simulink model "Prismatic_Power_Simulink"  (R2021a)
settings: Solver=VariableStepAuto  StartTime=0.0  StopTime=10.0  RelTol=1e-3
libraries: fl_lib x62, nesl_utility x24, fl_ps_legacy_lib x16, ee_lib x7, pid_lib x3, simulink x2
(part 1 of 2)
settings Model: Creator=Shivanshu  LastModifiedBy=Shivanshu

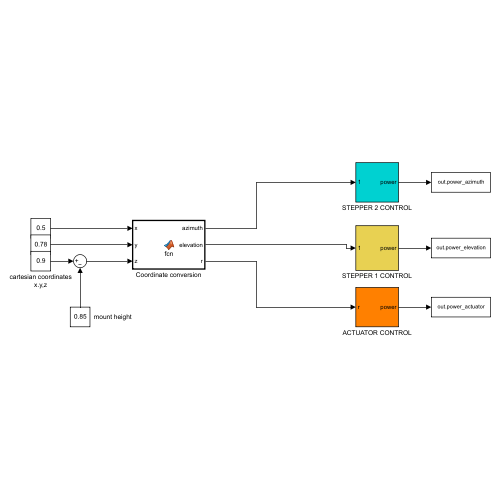
[thumbnail: Simulink's stored preview of the top-level diagram]
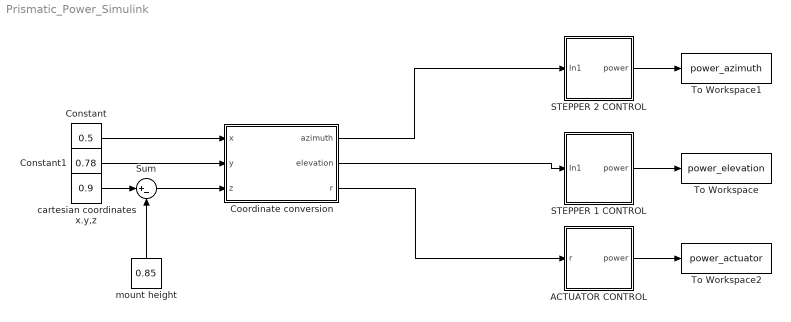
== system Prismatic_Power_Simulink ==
  ACTUATOR CONTROL : Subsystem  RequirementInfo={} %GIDa_0c115b90_ac6e_48f5_b72e_90011be317fb
  Constant : Constant  RequirementInfo={} %GIDa_f342d5e4_ff38_4643_bf1e_b5d7906d0ce5  Value=0.5
  Constant1 : Constant  RequirementInfo={} %GIDa_469f7adb_a8a1_4d2f_b1d5_d7893cc8c779  Value=0.78
  Coordinate conversion : MATLAB Function  RequirementInfo={} %GIDa_592b9090_c388_41e2_bff3_47ffeee67e9d  TreatAsAtomicUnit=on
  STEPPER 1 CONTROL : Subsystem  RequirementInfo={} %GIDa_0e8b4c65_2a77_43a1_8a22_c7e5a5acc945
  STEPPER 2 CONTROL : Subsystem  RequirementInfo={} %GIDa_86f44cae_780d_4682_ad09_b505177498bc
  Sum : Sum  Inputs=|+-
  To Workspace : ToWorkspace  VariableName=power_elevation  SampleTime=-1
  To Workspace1 : ToWorkspace  VariableName=power_azimuth  SampleTime=-1
  To Workspace2 : ToWorkspace  VariableName=power_actuator  SampleTime=-1
  cartesian coordinates x.y,z : Constant  RequirementInfo={} %GIDa_2cf69270_6584_4b69_8bd7_8d40a6ff0831  Value=0.9
  mount height : Constant  Value=0.85
  wires:
  Coordinate conversion/2(elevation) -> STEPPER 1 CONTROL/1(In1)
  Constant1/1 -> Coordinate conversion/2(y)
  Constant/1 -> Coordinate conversion/1(x)
  Coordinate conversion/1(azimuth) -> STEPPER 2 CONTROL/1(In1)
  Coordinate conversion/3(r) -> ACTUATOR CONTROL/1(r)
  Sum/1 -> Coordinate conversion/3(z)
  cartesian coordinates x.y,z/1 -> Sum/1
  mount height/1 -> Sum/2
  ACTUATOR CONTROL/1(power) -> To Workspace2/1
  STEPPER 1 CONTROL/1(power) -> To Workspace/1
  STEPPER 2 CONTROL/1(power) -> To Workspace1/1

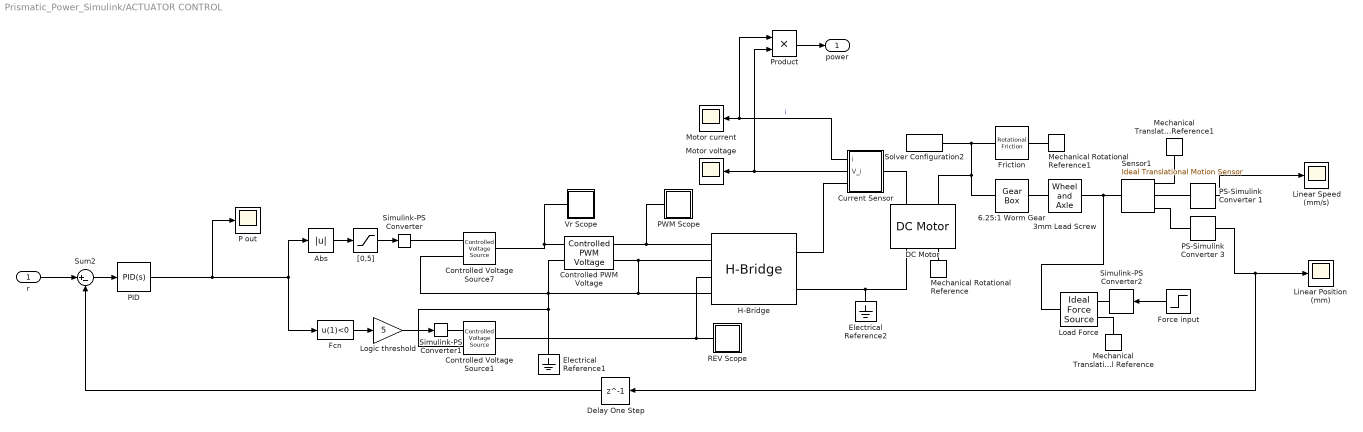
== system Prismatic_Power_Simulink/ACTUATOR CONTROL ==
  r : Inport  RequirementInfo={} %GIDa_01bbb075_66cd_4f10_a905_c743553500a9
  " PID" : pid_lib/PID Controller  RequirementInfo={} %GIDa_487d1a50_046a_4936_a3be_f4ba52b3f77b  Controller=PID  Form=Parallel  TimeDomain=Continuous-time  UseExternalTs=off  SampleTime=-1  IntegratorMethod=Forward Euler  FilterMethod=Forward Euler  ControllerParametersSource=internal  P=50  I=0  D=0  UseFilter=on  N=1  TunerSelectOption=Transfer Function Based (PID Tuner App)  InitialConditionSource=internal  InitialConditionForIntegrator=0  InitialConditionForFilter=0  DifferentiatorICPrevScaledInput=0  ExternalReset=none  TrackingMode=off  Kt=1  LimitOutput=off  SatLimitsSource=internal  UpperSaturationLimit=5  LowerSaturationLimit=-5  LinearizeAsGain=on  AntiWindupMode=back-calculation  Kb=1  POutMin=[]  POutMax=[]  IOutMin=[]  IOutMax=[]  DOutMin=[]  DOutMax=[]  NOutMin=[]  NOutMax=[]  SumOutMin=[]  SumOutMax=[]  SaturationOutMin=[]  SaturationOutMax=[]  PParamMin=[]  PParamMax=[]  IParamMin=[]  IParamMax=[]  DParamMin=[]  DParamMax=[]  NParamMin=[]  NParamMax=[]  KbParamMin=[]  KbParamMax=[]  KtParamMin=[]  KtParamMax=[]  KbOutMin=[]  KbOutMax=[]  KtOutMin=[]  KtOutMax=[]  IntegratorOutMin=[]  IntegratorOutMax=[]  FilterOutMin=[]  FilterOutMax=[]  SumI1OutMin=[]  SumI1OutMax=[]  SumI2OutMin=[]  SumI2OutMax=[]  SumI3OutMin=[]  SumI3OutMax=[]  SumI4OutMin=[]  SumI4OutMax=[]  SumDOutMin=[]  SumDOutMax=[]  DifferentiatorOutMin=[]  DifferentiatorOutMax=[]  FilterDiffOutCoefMin=[]  FilterDiffOutCoefMax=[]  ReciprocalOutMin=[]  ReciprocalOutMax=[]  SumDenOutMin=[]  SumDenOutMax=[]  SumNumOutMin=[]  SumNumOutMax=[]  DivideOutMin=[]  DivideOutMax=[]  UdiffTsProdOutMin=[]  UdiffTsProdOutMax=[]  NTsProdOutMin=[]  NTsProdOutMax=[]  UintegralTsProdOutMin=[]  UintegralTsProdOutMax=[]  UngainTsProdOutMin=[]  UngainTsProdOutMax=[]  IntegratorContinuousStateAttributes=''  IntegratorStateMustResolveToSignalObject=off  IntegratorRTWStateStorageClass=Auto  FilterContinuousStateAttributes=''  FilterStateMustResolveToSignalObject=off  FilterRTWStateStorageClass=Auto  ParallelPVariant=InternalParameters  IdealPVariant=Disabled  IVariant=InternalParameters  DVariant=InternalParameters  IntegratorVariant=Continuous  SatVariant=Disabled  AWVariant=Passthrough  PCopyVariant=Disabled  TRVariant=Disabled  FdbkBlocksVariant=Forward  IdealPFdbkVariant=Disabled  SatFdbkVariant=Disabled  DerivativeFilterVariant=ContFilter  NVariant=InternalParameters  NCopyVariant=Disabled  FilterICVariant=InternalICsFilter  IntegratorICVariant=InternalICs  ExternalResetVariant=Disabled  TRSumVariant=Passthrough  SumFdbkVariant=Disabled  SumVariant=Sum_PID  TsampFilterVariant=InternalTs  TsampNgainVariant=Passthrough  TsampIntegralVariant=Passthrough  ExternalSaturationOutDataTypeStr=Inherit: Same as second input
  3mm Lead Screw : fl_lib/Mechanical/Mechanisms/Wheel and Axle  RequirementInfo={} %GIDa_63769a3e_da90_4985_9ff6_81674143f087  R=3e-3/(2*pi) m  or=1  t_specify=off  t_priority=High  t=0 N*m  t_nominal_specify=off  t_nominal_unit=N*m  t_nominal_value=1  f_specify=off  f_priority=High  f=0 N  f_nominal_specify=off  f_nominal_unit=N  f_nominal_value=1
  6.25:1 Worm Gear : fl_lib/Mechanical/Mechanisms/Gear Box  RequirementInfo={} %GIDa_72538fa4_a052_4650_b0d0_d2ddea2e6bef  ratio=1  t_in_specify=off  t_in_priority=High  t_in=0 N*m  t_in_nominal_specify=off  t_in_nominal_unit=N*m  t_in_nominal_value=1  t_out_specify=off  t_out_priority=High  t_out=0 N*m  t_out_nominal_specify=off  t_out_nominal_unit=N*m  t_out_nominal_value=1
  Abs : Abs  RequirementInfo={} %GIDa_f6d84932_f9cc_4ae6_b8c7_05faab76c6e2
  Controlled PWM Voltage : ee_lib/Integrated Circuits/Controlled PWM Voltage  RequirementInfo={} %GIDa_27007e47_f5f5_44e8_a6b6_33ad898611cc  F=10000 Hz  TD=0 s  pulse_width_offset=0 s  pulse_min=0 s  pwm_or_av=2  event_type=1  sample_time=1e-6 s  Vmin=0 V  Vmax=5 V  Vm=5 V  u_min=0  u_max=1
  Controlled Voltage Source1 : fl_lib/Electrical/Electrical Sources/Controlled Voltage Source
  Controlled Voltage Source7 : fl_lib/Electrical/Electrical Sources/Controlled Voltage Source
  Current Sensor : Subsystem  RequirementInfo={} %GIDa_951e5fb8_fda0_4450_be3e_49b1b835e176
  DC Motor : ee_lib/Electromechanical/Brushed Motors/DC Motor  RequirementInfo={} %GIDa_7affa033_7e69_4159_88fa_8fc21d2e6eba  field_option=ee.enum.field_option.pm  Rf=100 Ohm  Lf=1 H  Laf=0.15 H  If0=0 A  parameterization=1  Ra=4.8 Ohm  La=1600e-6 H  emf_or_torque=2  Kv=0.0637 V/rpm  Ki=0.0637 N*m/A  T_stall=3e-3*4000/(2*pi*6.25) N*m  w_max=3250 rpm  w_rated=2375 rpm  P_rated=19 W  V_rated=24 V  lam_param=1  i_noload=0 A  V_i_noload=1.5 V  J=2.5e-5 kg*m^2  lam=1e-08 N*m/(rad/s)  speed0=0 rpm  enable_fault_armature=simscape.enum.onoff.off  rev_faulted=1 / 3  G_faulted_armature=1e-5 S  fault_trigger_armature=ee.enum.faults.faultTrigger.temporal  t_fault_armature=1 s  max_permissible_current_armature=inf A  t_fail_on_current_armature=1 s  enable_fault_field=simscape.enum.onoff.off  G_faulted_field=1e-5 S  fault_trigger_field=ee.enum.faults.faultTrigger.temporal  t_fault_field=1 s  max_permissible_current_field=inf A  t_fail_on_current_field=1 s  fault_action=simscape.enum.assert.action.none  alpha=3.93e-3 1/K  Tmeas=25 degC  thermal_mass=100 J/K  initial_temperature=25 degC
  Delay One Step : Delay  DelayLength=1
  Electrical Reference1 : fl_lib/Electrical/Electrical Elements/Electrical Reference  RequirementInfo={} %GIDa_89b08f27_1c28_43fa_90f1_c3e1b2523f66
  Electrical Reference2 : fl_lib/Electrical/Electrical Elements/Electrical Reference  RequirementInfo={} %GIDa_89f9a18e_2c45_4337_9d4e_60fab91f8798
  Fcn : Fcn  RequirementInfo={} %GIDa_e3655066_669c_45fb_9a19_17bddf37387a  Expr=u(1)<0
  Force input : Step  RequirementInfo={} %GIDa_8bd74132_84d7_49a1_938c_4321d642dd77  Time=0  After=26  SampleTime=0
  Friction : fl_lib/Mechanical/Rotational Elements/Rotational Friction  RequirementInfo={} %GIDa_e06c0b92_9617_4ed0_a579_d175118991af  brkwy_trq=3.0e-2 N*m  brkwy_vel=0.03347 rad/s  Col_trq=3.0e-2 N*m  visc_coef=0 N*m/(rad/s)  w_specify=off  w_priority=High  w=0 rad/s  w_nominal_specify=off  w_nominal_unit=rad/s  w_nominal_value=1  t_specify=off  t_priority=High  t=0 N*m  t_nominal_specify=off  t_nominal_unit=N*m  t_nominal_value=1
  H-Bridge : ee_lib/Semiconductors & Converters/Converters/H-Bridge  RequirementInfo={} %GIDa_56669dc1_63b8_4cf5_93b6_3c8bc310ad95  supply_ports=ee.enum.supply_ports.hidesupply  pwm_or_av=2  regenerative_braking_mode=ee.enum.converters.regenerative_braking_mode.depends_on_rev  discontinuous=0  freewheeling_mode=1  Rload=10 Ohm  Lload=1e-5 H  F=10 kHz  Venable=2.5 V  Vmax=5 V  Vreverse=2.5 V  Vbrake=2.5 V  Vm=24 V  Ron=0.1 Ohm  Don=0.1 Ohm  Goff=1e-6 S  Tmeas=298.15 K  Ron2=0.1 Ohm  Don2=0.05 Ohm  Tmeas2=398.15 K  thermal_mass=100 J/K  initial_temperature=298.15 K
  Linear Position (mm) : Scope
      settings: RequirementInfo={} %GIDa_41f36c91_7ebd_4c66_9021_a254624060f4
  Linear Speed (mm/s) : Scope
      settings: RequirementInfo={} %GIDa_e7e46648_1c56_4b94_9344_d70892eaff83
  Load Force : fl_lib/Mechanical/Mechanical Sources/Ideal Force Source
  Logic threshold : Gain  RequirementInfo={} %GIDa_1909a90c_10d8_48a1_af66_de6e9db6703c  Gain=5
  Mechanical Rotational Reference : fl_lib/Mechanical/Rotational Elements/Mechanical Rotational Reference  RequirementInfo={} %GIDa_63f71ed3_fef8_4f75_98eb_8c5a89edb114
  Mechanical Rotational Reference1 : fl_lib/Mechanical/Rotational Elements/Mechanical Rotational Reference  RequirementInfo={} %GIDa_5e27ac28_5aaf_4b31_8da8_b6d3661061ca
  Mechanical Translational Reference : fl_lib/Mechanical/Translational Elements/Mechanical Translational Reference
  Mechanical Translational Reference1 : fl_lib/Mechanical/Translational Elements/Mechanical Translational Reference  RequirementInfo={} %GIDa_7d591b10_55f0_4606_80de_d7dbcf0dd33a
  Motor current : Scope
      settings: RequirementInfo={} %GIDa_bc7ecbe7_9427_4297_b096_91eef305f549
  Motor voltage : Scope
  P out : Scope
      settings: RequirementInfo={} %GIDa_dbff9b42_3c0c_4d19_b1f1_d04575505001
  PS-Simulink Converter 1 : nesl_utility/PS-Simulink Converter  RequirementInfo={} %GIDa_15f4e04d_f060_4352_858a_10e846c21cdf  PhysicalDomain=network_engine_domain  SubClassName=ps_output  LeftPortType=input  RightPortType=output  PseudoPeriodic=off  Frequencies=[]  Unit=mm/s  AffineConversion=off
      settings: SourceProductBaseCode=PW,SS
  PS-Simulink Converter 3 : nesl_utility/PS-Simulink Converter  RequirementInfo={} %GIDa_30ed7d89_fbbb_4963_8d8f_8bdecd8b3340  PhysicalDomain=network_engine_domain  SubClassName=ps_output  LeftPortType=input  RightPortType=output  PseudoPeriodic=off  Frequencies=[]  Unit=mm  AffineConversion=off
      settings: SourceProductBaseCode=PW,SS
  PWM Scope : Subsystem  RequirementInfo={} %GIDa_efacd876_f880_4d28_9dde_cc613583df43
  Product : Product
  REV Scope : Subsystem  RequirementInfo={} %GIDa_f2ecff02_609c_450c_8d23_0624da6bc12d
  Sensor1 : fl_lib/Mechanical/Mechanical Sensors/Ideal Translational Motion Sensor  RequirementInfo={} %GIDa_c8600ff7_c347_4738_a653_ffa1c1e64037  offset=0 m
  Simulink-PS Converter : nesl_utility/Simulink-PS Converter  PhysicalDomain=network_engine_domain  SubClassName=ps_input  LeftPortType=input  RightPortType=output  PseudoPeriodic=off  Frequencies=[]  NoiseDistribution=none  NoiseParameters=[]  Unit=1  AffineConversion=off  FilteringAndDerivatives=provide  SimscapeFilterOrder=1  InputFilterTimeConstant=0.001  UdotUserProvided=0
      settings: SourceProductBaseCode=PW,SS
  Simulink-PS Converter1 : nesl_utility/Simulink-PS Converter  PhysicalDomain=network_engine_domain  SubClassName=ps_input  LeftPortType=input  RightPortType=output  PseudoPeriodic=off  Frequencies=[]  NoiseDistribution=none  NoiseParameters=[]  Unit=1  AffineConversion=off  FilteringAndDerivatives=provide  SimscapeFilterOrder=1  InputFilterTimeConstant=0.001  UdotUserProvided=0
      settings: SourceProductBaseCode=PW,SS
  Simulink-PS Converter2 : nesl_utility/Simulink-PS Converter  PhysicalDomain=network_engine_domain  SubClassName=ps_input  LeftPortType=input  RightPortType=output  PseudoPeriodic=off  Frequencies=[]  NoiseDistribution=none  NoiseParameters=[]  Unit=N  AffineConversion=off  FilteringAndDerivatives=zero  SimscapeFilterOrder=1  InputFilterTimeConstant=.001  UdotUserProvided=0
      settings: SourceProductBaseCode=PW,SS
  Solver Configuration2 : nesl_utility/Solver Configuration  RequirementInfo={} %GIDa_e47c6a6f_f974_48ac_ab36_2c055cf36617  PhysicalDomain=network_engine_domain  SubClassName=solver  LeftPortType=input  RightPortType=generic  Tones=[]  Harmonics=[]  SimulateNoise=off  Profile=off  UseLocalSampling=off  EnableSwitchedLinearOptims=on  FrequencyDomain=off  UseCCode=off  RelTol=0.001  AbsTol=1e-06  MinStep=1e-09  ToWorkspace=off  RevertToSquareIcSolve=off  NumHomotopyIterations=100  PhasorMode=off  PhasorModeNumHarmonics=1  DoDC=off  ResidualTolerance=1e-7  UseLocalSolver=off  LocalSolverChoice=NE_BACKWARD_EULER_ADVANCER  LocalSolverSampleTime=.001  DoFixedCost=off  MaxNonlinIter=3  MaxModeIter=2  ComputeImpulses=off  ImpulseIterations=2  LinearAlgebra=Sparse  EquationFormulation=NE_TIME_EF  DelaysMemoryBudget=1024  AutomaticFiltering=on  FilteringTimeConstant=0.001  PartitionStorageMethod=AS_NEEDED  PartitionMemoryBudget=1024  PartitionMethod=FAST
      settings: SourceProductBaseCode=PW,SS
  Sum2 : Sum  RequirementInfo={} %GIDa_e5c6e740_0488_4797_a1b9_c712b45697aa  Inputs=|+-
  Vr Scope : Subsystem  RequirementInfo={} %GIDa_855e83c9_6e95_4328_8826_9e2a8425f04e
  "[0,5]" : Saturate  RequirementInfo={} %GIDa_3688256d_56e0_4fa1_a257_885808f5b2d2  UpperLimit=5  LowerLimit=0
  power : Outport
  wires:
  Sum2/1 -> " PID"/1
  PS-Simulink Converter 3/1 -> Delay One Step/1, Linear Position (mm)/1
  Logic threshold/1 -> Simulink-PS Converter1/1
  Fcn/1 -> Logic threshold/1
  Abs/1 -> "[0,5]"/1
  " PID"/1 -> Abs/1, Fcn/1, P out/1
  r/1 -> Sum2/1
  PS-Simulink Converter 1/1 -> Linear Speed (mm/s)/1
  Current Sensor/1(i) -> Product/1, Motor current/1  "i"
  "[0,5]"/1 -> Simulink-PS Converter/1
  Force input/1 -> Simulink-PS Converter2/1
  Current Sensor/2(V_i) -> Product/2, Motor voltage/1
  Product/1 -> power/1
  Delay One Step/1 -> Sum2/2
  connections:
  Sensor1/RConn3 -- PS-Simulink Converter 3/LConn1
  6.25:1 Worm Gear/RConn1 -- 3mm Lead Screw/LConn1
  Sensor1/RConn2 -- PS-Simulink Converter 1/LConn1
  DC Motor/RConn2 -- Mechanical Rotational Reference/LConn1
  Friction/LConn1 -- 6.25:1 Worm Gear/LConn1 -- DC Motor/LConn2 -- Solver Configuration2/RConn1
  3mm Lead Screw/RConn1 -- Load Force/LConn1 -- Sensor1/LConn1
  Sensor1/RConn1 -- Mechanical Translational Reference1/LConn1
  Mechanical Rotational Reference1/LConn1 -- Friction/RConn1
  Current Sensor/LConn1 -- DC Motor/LConn1
  H-Bridge/LConn3 -- Controlled Voltage Source1/LConn1 -- REV Scope/LConn1
  Controlled PWM Voltage/LConn1 -- Vr Scope/LConn1 -- Controlled Voltage Source7/LConn1
  Controlled PWM Voltage/RConn1 -- PWM Scope/LConn1 -- H-Bridge/LConn1
  Controlled PWM Voltage/RConn2 -- H-Bridge/LConn2 -- Controlled Voltage Source1/RConn2 -- Electrical Reference1/LConn1 -- Controlled Voltage Source7/RConn2 -- Controlled PWM Voltage/LConn2 -- H-Bridge/LConn4
  H-Bridge/RConn2 -- DC Motor/RConn1 -- Electrical Reference2/LConn1
  Current Sensor/RConn1 -- H-Bridge/RConn1
  Simulink-PS Converter/RConn1 -- Controlled Voltage Source7/RConn1
  Controlled Voltage Source1/RConn1 -- Simulink-PS Converter1/RConn1
  Load Force/RConn2 -- Mechanical Translational Reference/LConn1
  Load Force/RConn1 -- Simulink-PS Converter2/RConn1

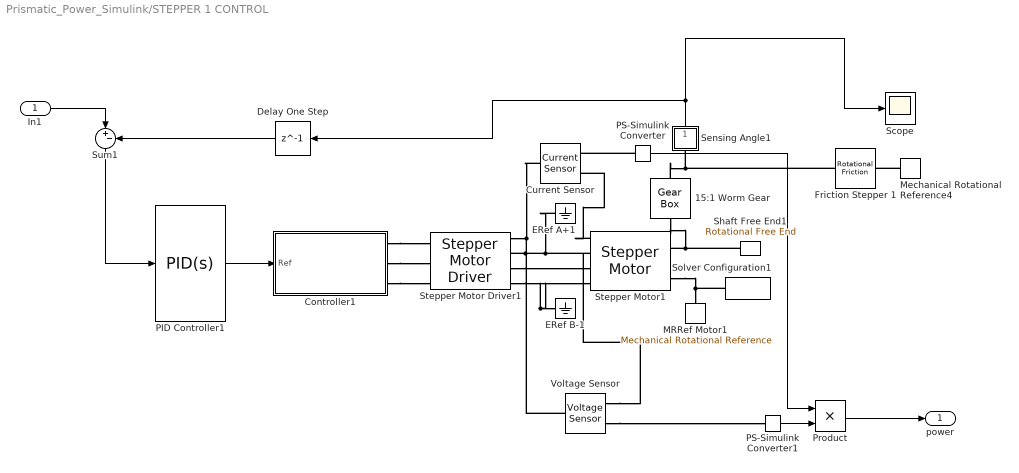
== system Prismatic_Power_Simulink/STEPPER 1 CONTROL ==
  In1 : Inport  RequirementInfo={} %GIDa_e169cb36_29c5_44db_b81c_ecb589be7782
  15:1 Worm Gear : fl_lib/Mechanical/Mechanisms/Gear Box  ratio=1/15  t_in_specify=off  t_in_priority=High  t_in=0 N*m  t_in_nominal_specify=off  t_in_nominal_unit=N*m  t_in_nominal_value=1  t_out_specify=off  t_out_priority=High  t_out=0 N*m  t_out_nominal_specify=off  t_out_nominal_unit=N*m  t_out_nominal_value=1
  Controller1 : Subsystem  RequirementInfo={} %GIDa_f5243d20_398c_4fff_b1cc_7e92ed00deb8  Variant=on  VariantControlMode=label  LabelModeActiveChoice=Speed
      settings: AttributesFormatString=%<BlockChoice>
  Current Sensor : fl_lib/Electrical/Electrical Sensors/Current Sensor
  Delay One Step : Delay  DelayLength=1
  ERef A+1 : fl_lib/Electrical/Electrical Elements/Electrical Reference  RequirementInfo={} %GIDa_91f8b646_79cb_4fea_bb0d_768587617fa3
  ERef B-1 : fl_lib/Electrical/Electrical Elements/Electrical Reference  RequirementInfo={} %GIDa_dce07608_cfc0_4bcf_a795_dd87c59b02fd
  Friction Stepper 1 : fl_lib/Mechanical/Rotational Elements/Rotational Friction  RequirementInfo={} %GIDa_8d335118_6bb8_4449_8481_e559c0f05eb6  brkwy_trq=3.0e-2 N*m  brkwy_vel=0.03347 rad/s  Col_trq=3.0e-2 N*m  visc_coef=0 N*m/(rad/s)  w_specify=off  w_priority=High  w=0 rad/s  w_nominal_specify=off  w_nominal_unit=rad/s  w_nominal_value=1  t_specify=off  t_priority=High  t=0 N*m  t_nominal_specify=off  t_nominal_unit=N*m  t_nominal_value=1
  MRRef Motor1 : fl_lib/Mechanical/Rotational Elements/Mechanical Rotational Reference  RequirementInfo={} %GIDa_c279d1ab_3163_46c3_8afc_72e7a25ed2f5
  Mechanical Rotational Reference4 : fl_lib/Mechanical/Rotational Elements/Mechanical Rotational Reference  RequirementInfo={} %GIDa_816df603_38fd_454e_955f_a2f0381ebda9
  PID Controller1 : pid_lib/PID Controller  RequirementInfo={} %GIDa_a31db279_d66f_471e_a906_b25fbe89d565  Controller=PID  Form=Parallel  TimeDomain=Continuous-time  UseExternalTs=off  SampleTime=-1  IntegratorMethod=Forward Euler  FilterMethod=Forward Euler  ControllerParametersSource=internal  P=6  I=6  D=0  UseFilter=on  N=100  TunerSelectOption=Transfer Function Based (PID Tuner App)  InitialConditionSource=internal  InitialConditionForIntegrator=0  InitialConditionForFilter=0  DifferentiatorICPrevScaledInput=0  ExternalReset=none  TrackingMode=off  Kt=1  LimitOutput=off  SatLimitsSource=internal  UpperSaturationLimit=inf  LowerSaturationLimit=-inf  LinearizeAsGain=on  AntiWindupMode=none  Kb=1  POutMin=[]  POutMax=[]  IOutMin=[]  IOutMax=[]  DOutMin=[]  DOutMax=[]  NOutMin=[]  NOutMax=[]  SumOutMin=[]  SumOutMax=[]  SaturationOutMin=[]  SaturationOutMax=[]  PParamMin=[]  PParamMax=[]  IParamMin=[]  IParamMax=[]  DParamMin=[]  DParamMax=[]  NParamMin=[]  NParamMax=[]  KbParamMin=[]  KbParamMax=[]  KtParamMin=[]  KtParamMax=[]  KbOutMin=[]  KbOutMax=[]  KtOutMin=[]  KtOutMax=[]  IntegratorOutMin=[]  IntegratorOutMax=[]  FilterOutMin=[]  FilterOutMax=[]  SumI1OutMin=[]  SumI1OutMax=[]  SumI2OutMin=[]  SumI2OutMax=[]  SumI3OutMin=[]  SumI3OutMax=[]  SumI4OutMin=[]  SumI4OutMax=[]  SumDOutMin=[]  SumDOutMax=[]  DifferentiatorOutMin=[]  DifferentiatorOutMax=[]  FilterDiffOutCoefMin=[]  FilterDiffOutCoefMax=[]  ReciprocalOutMin=[]  ReciprocalOutMax=[]  SumDenOutMin=[]  SumDenOutMax=[]  SumNumOutMin=[]  SumNumOutMax=[]  DivideOutMin=[]  DivideOutMax=[]  UdiffTsProdOutMin=[]  UdiffTsProdOutMax=[]  NTsProdOutMin=[]  NTsProdOutMax=[]  UintegralTsProdOutMin=[]  UintegralTsProdOutMax=[]  UngainTsProdOutMin=[]  UngainTsProdOutMax=[]  IntegratorContinuousStateAttributes=''  IntegratorStateMustResolveToSignalObject=off  IntegratorRTWStateStorageClass=Auto  FilterContinuousStateAttributes=''  FilterStateMustResolveToSignalObject=off  FilterRTWStateStorageClass=Auto  ParallelPVariant=InternalParameters  IdealPVariant=Disabled  IVariant=InternalParameters  DVariant=InternalParameters  IntegratorVariant=Continuous  SatVariant=Disabled  AWVariant=Passthrough  PCopyVariant=Disabled  TRVariant=Disabled  FdbkBlocksVariant=Forward  IdealPFdbkVariant=Disabled  SatFdbkVariant=Disabled  DerivativeFilterVariant=ContFilter  NVariant=InternalParameters  NCopyVariant=Disabled  FilterICVariant=InternalICsFilter  IntegratorICVariant=InternalICs  ExternalResetVariant=Disabled  TRSumVariant=Passthrough  SumFdbkVariant=Disabled  SumVariant=Sum_PID  TsampFilterVariant=InternalTs  TsampNgainVariant=Passthrough  TsampIntegralVariant=Passthrough  ExternalSaturationOutDataTypeStr=Inherit: Same as second input
  PS-Simulink Converter : nesl_utility/PS-Simulink Converter  PhysicalDomain=network_engine_domain  SubClassName=ps_output  LeftPortType=input  RightPortType=output  PseudoPeriodic=off  Frequencies=[]  Unit=inherit  AffineConversion=off
      settings: SourceProductBaseCode=PW,SS
  PS-Simulink Converter1 : nesl_utility/PS-Simulink Converter  PhysicalDomain=network_engine_domain  SubClassName=ps_output  LeftPortType=input  RightPortType=output  PseudoPeriodic=off  Frequencies=[]  Unit=inherit  AffineConversion=off
      settings: SourceProductBaseCode=PW,SS
  Product : Product
  Scope : Scope
      settings: RequirementInfo={} %GIDa_4a877b93_832a_4353_b61a_570bc3f97895
  Sensing Angle1 : Subsystem  RequirementInfo={} %GIDa_0b6daea7_90cf_4cdb_bcc7_c201abae979b
      mask Display: disp('a')
  Shaft Free End1 : fl_lib/Mechanical/Rotational Elements/Rotational Free End  RequirementInfo={} %GIDa_a996d801_e28b_4806_adaf_abaf85496fa5  w_specify=off  w_priority=None  w=0 rad/s  w_nominal_specify=off  w_nominal_unit=rad/s  w_nominal_value=1
      settings: SourceProductBaseCode=SS
  Solver Configuration1 : nesl_utility/Solver Configuration  RequirementInfo={} %GIDa_18c0e3bd_09ef_420e_8c7d_4c14b245c5e2  PhysicalDomain=network_engine_domain  SubClassName=solver  LeftPortType=input  RightPortType=generic  Tones=[]  Harmonics=[]  SimulateNoise=off  Profile=off  UseLocalSampling=off  EnableSwitchedLinearOptims=on  FrequencyDomain=off  UseCCode=off  RelTol=0.001  AbsTol=1e-06  MinStep=1e-09  ToWorkspace=off  RevertToSquareIcSolve=off  NumHomotopyIterations=100  PhasorMode=off  PhasorModeNumHarmonics=1  DoDC=off  ResidualTolerance=1e-7  UseLocalSolver=off  LocalSolverChoice=NE_BACKWARD_EULER_ADVANCER  LocalSolverSampleTime=.001  DoFixedCost=off  MaxNonlinIter=3  MaxModeIter=2  ComputeImpulses=off  ImpulseIterations=2  LinearAlgebra=auto  EquationFormulation=NE_TIME_EF  DelaysMemoryBudget=1024  AutomaticFiltering=on  FilteringTimeConstant=0.001  PartitionStorageMethod=AS_NEEDED  PartitionMemoryBudget=1024  PartitionMethod=FAST
      settings: SourceProductBaseCode=PW,SS
  Stepper Motor Driver1 : ee_lib/Electromechanical/Reluctance & Stepper/Stepper Motor Driver  RequirementInfo={} %GIDa_af48d62f_cdf6_4fd4_9765_69e953716fad  step_or_av=ee.enum.electromech.simulationMode.stepping  step_rate_per_volt=10 Hz/V  Venable=2.5 V  Vreverse=2.5 V  supply_ports=ee.enum.supply_ports.hidesupply  Vm=5 V  Vsupply=10 V  half_stepping=ee.enum.electromech.steppingModeAveraged.fullStep  stepping_mode=ee.enum.electromech.steppingMode.microStep  numMicroSteps=4  Im=1.2 A
      settings: SourceProductBaseCode=PS  InternalSimscapePortConfiguration="{\"Bottom\":[],\"Left\":[{\"id\":\"ENA\",\"label\":\"ENA\",\"type\":\"foundation.electrical.electrical\"},{\"id\":\"REF\",\"label\":\"REF\",\"type\":\"foundation.electrical.electrical\"},{\"id\":\"REV\",\"label\":\"REV\",\"type\":\"foundation.electrical.electrical\"}],\"Right\":[{\"id\":\"pA\",\"label\":\"A+\",\"type\":\"foundation.electrical.electrical\"},{\"id\":\"nA\",\"label\":\"A-\",\"type\":\"foundation.electrical.electrical\"},{\"id\":\"pB\",\"label\":\"B+\",\"type\":\"foundation.electrical.electrical\"},{\"id\":\"nB\",\"label\":\"B-\",\"type\":\"foundation.electrical.electrical\"}],\"Top\":[]}"
  Stepper Motor1 : ee_lib/Electromechanical/Reluctance & Stepper/Stepper Motor  RequirementInfo={} %GIDa_733456ab_00aa_45b3_baab_6baf17ab8f3f  step_or_av=ee.enum.electromech.simulationMode.stepping  Ra=0.35 Ohm  La=1.8 mH  Km=0.678 N*m/A  Td=0.065 N*m  Rm=Inf Ohm  w_vec=[ 0 1000 3e+3 ] rpm  T_vec=[ 2 2 1 ] N*m  assert_if_slipping=ee.enum.assertAction.none  J_total=1e-4 kg*m^2  max_step_rate=10 Hz  Step=1.8 deg  J=480 g*cm^2  B=1e-02 N*m/(rad/s)  speed0=0 rpm  theta0=0 deg  alpha=[.00393, .00393] 1/K  Tmeas=25 degC  Tmeas2=125 degC  T_vec2=[1.7, 1.7, .85] N*m  half_stepping=ee.enum.electromech.steppingModeAveraged.fullStep  thermal_masses=[100, 100] J/K  initial_temperatures=[25, 25] degC  rotor_thermal_mass=50 J/K  rotor_initial_temperature=25 degC  Rm_percent_rotor=90
      settings: SourceProductBaseCode=PS  InternalSimscapePortConfiguration="{\"Bottom\":[],\"Left\":[{\"id\":\"pA\",\"label\":\"A+\",\"type\":\"foundation.electrical.electrical\"},{\"id\":\"nA\",\"label\":\"A-\",\"type\":\"foundation.electrical.electrical\"},{\"id\":\"pB\",\"label\":\"B+\",\"type\":\"foundation.electrical.electrical\"},{\"id\":\"nB\",\"label\":\"B-\",\"type\":\"foundation.electrical.electrical\"}],\"Right\":[{\"id\":\"R\",\"label\":\"R\",\"type\":\"foundation.mechanical.rotational.rotational\"},{\"id\":\"C\",\"label\":\"C\",\"type\":\"foundation.mechanical.rotational.rotational\"}],\"Top\":[]}"
  Sum1 : Sum  RequirementInfo={} %GIDa_a9460d84_32fc_41ef_955c_7c410545f0e3  Inputs=|+-
  Voltage Sensor : fl_lib/Electrical/Electrical Sensors/Voltage Sensor
  power : Outport
  wires:
  Sum1/1 -> PID Controller1/1
  Sensing Angle1/1(theta) -> Delay One Step/1, Scope/1
  In1/1 -> Sum1/1
  PID Controller1/1 -> Controller1/1(Ref)
  PS-Simulink Converter/1 -> Product/1
  Product/1 -> power/1
  PS-Simulink Converter1/1 -> Product/2
  Delay One Step/1 -> Sum1/2
  connections:
  Stepper Motor Driver1/RConn3 -- Stepper Motor1/LConn3
  Controller1/RConn1 -- Stepper Motor Driver1/LConn1
  MRRef Motor1/LConn1 -- Stepper Motor1/RConn2 -- Solver Configuration1/RConn1
  Controller1/RConn3 -- Stepper Motor Driver1/LConn3
  Mechanical Rotational Reference4/LConn1 -- Friction Stepper 1/RConn1
  Friction Stepper 1/LConn1 -- 15:1 Worm Gear/RConn1 -- Sensing Angle1/LConn1
  ERef B-1/LConn1 -- Stepper Motor Driver1/RConn4 -- Stepper Motor1/LConn4
  Stepper Motor Driver1/RConn2 -- Voltage Sensor/RConn2 -- Stepper Motor1/LConn2 -- ERef A+1/LConn1
  Controller1/RConn2 -- Stepper Motor Driver1/LConn2
  Stepper Motor Driver1/RConn1 -- Current Sensor/LConn1 -- Voltage Sensor/LConn1
  Shaft Free End1/LConn1 -- 15:1 Worm Gear/LConn1 -- Stepper Motor1/RConn1
  Voltage Sensor/RConn1 -- PS-Simulink Converter1/LConn1
  PS-Simulink Converter/LConn1 -- Current Sensor/RConn1
  Stepper Motor1/LConn1 -- Current Sensor/RConn2

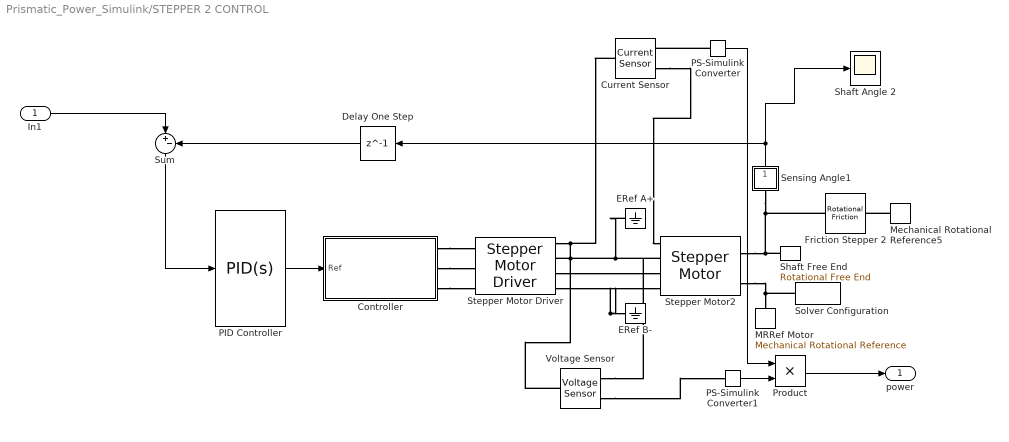
== system Prismatic_Power_Simulink/STEPPER 2 CONTROL ==
  In1 : Inport  RequirementInfo={} %GIDa_4d72656e_6302_4bc2_9162_a0a21af42942
  Controller : Subsystem  RequirementInfo={} %GIDa_7fa7e0dc_6309_48d9_905c_56e801f25fe6  Variant=on  VariantControlMode=label  LabelModeActiveChoice=Speed
      settings: AttributesFormatString=%<BlockChoice>
  Current Sensor : fl_lib/Electrical/Electrical Sensors/Current Sensor
  Delay One Step : Delay  DelayLength=1
  ERef A+ : fl_lib/Electrical/Electrical Elements/Electrical Reference  RequirementInfo={} %GIDa_0ed44354_a11b_4d70_9a75_5aceded45322
  ERef B- : fl_lib/Electrical/Electrical Elements/Electrical Reference  RequirementInfo={} %GIDa_b34c45eb_08ce_44cf_9e33_e2c98d20e31b
  Friction Stepper 2 : fl_lib/Mechanical/Rotational Elements/Rotational Friction  RequirementInfo={} %GIDa_067ecdbb_d6db_41c9_a42c_f5e57237fa42  brkwy_trq=3.0e-2 N*m  brkwy_vel=0.03347 rad/s  Col_trq=3.0e-2 N*m  visc_coef=0 N*m/(rad/s)  w_specify=off  w_priority=High  w=0 rad/s  w_nominal_specify=off  w_nominal_unit=rad/s  w_nominal_value=1  t_specify=off  t_priority=High  t=0 N*m  t_nominal_specify=off  t_nominal_unit=N*m  t_nominal_value=1
  MRRef Motor : fl_lib/Mechanical/Rotational Elements/Mechanical Rotational Reference  RequirementInfo={} %GIDa_61bcd8c5_289e_4c53_9e68_7ec84301093f
  Mechanical Rotational Reference5 : fl_lib/Mechanical/Rotational Elements/Mechanical Rotational Reference  RequirementInfo={} %GIDa_c9921306_9976_4945_890f_c483cce1d17d
  PID Controller : pid_lib/PID Controller  RequirementInfo={} %GIDa_45716794_6d57_4096_b132_e32ca8f6ff4f  Controller=PID  Form=Parallel  TimeDomain=Continuous-time  UseExternalTs=off  SampleTime=-1  IntegratorMethod=Forward Euler  FilterMethod=Forward Euler  ControllerParametersSource=internal  P=6  I=6  D=0  UseFilter=on  N=100  TunerSelectOption=Transfer Function Based (PID Tuner App)  InitialConditionSource=internal  InitialConditionForIntegrator=0  InitialConditionForFilter=0  DifferentiatorICPrevScaledInput=0  ExternalReset=none  TrackingMode=off  Kt=1  LimitOutput=off  SatLimitsSource=internal  UpperSaturationLimit=inf  LowerSaturationLimit=-inf  LinearizeAsGain=on  AntiWindupMode=none  Kb=1  POutMin=[]  POutMax=[]  IOutMin=[]  IOutMax=[]  DOutMin=[]  DOutMax=[]  NOutMin=[]  NOutMax=[]  SumOutMin=[]  SumOutMax=[]  SaturationOutMin=[]  SaturationOutMax=[]  PParamMin=[]  PParamMax=[]  IParamMin=[]  IParamMax=[]  DParamMin=[]  DParamMax=[]  NParamMin=[]  NParamMax=[]  KbParamMin=[]  KbParamMax=[]  KtParamMin=[]  KtParamMax=[]  KbOutMin=[]  KbOutMax=[]  KtOutMin=[]  KtOutMax=[]  IntegratorOutMin=[]  IntegratorOutMax=[]  FilterOutMin=[]  FilterOutMax=[]  SumI1OutMin=[]  SumI1OutMax=[]  SumI2OutMin=[]  SumI2OutMax=[]  SumI3OutMin=[]  SumI3OutMax=[]  SumI4OutMin=[]  SumI4OutMax=[]  SumDOutMin=[]  SumDOutMax=[]  DifferentiatorOutMin=[]  DifferentiatorOutMax=[]  FilterDiffOutCoefMin=[]  FilterDiffOutCoefMax=[]  ReciprocalOutMin=[]  ReciprocalOutMax=[]  SumDenOutMin=[]  SumDenOutMax=[]  SumNumOutMin=[]  SumNumOutMax=[]  DivideOutMin=[]  DivideOutMax=[]  UdiffTsProdOutMin=[]  UdiffTsProdOutMax=[]  NTsProdOutMin=[]  NTsProdOutMax=[]  UintegralTsProdOutMin=[]  UintegralTsProdOutMax=[]  UngainTsProdOutMin=[]  UngainTsProdOutMax=[]  IntegratorContinuousStateAttributes=''  IntegratorStateMustResolveToSignalObject=off  IntegratorRTWStateStorageClass=Auto  FilterContinuousStateAttributes=''  FilterStateMustResolveToSignalObject=off  FilterRTWStateStorageClass=Auto  ParallelPVariant=InternalParameters  IdealPVariant=Disabled  IVariant=InternalParameters  DVariant=InternalParameters  IntegratorVariant=Continuous  SatVariant=Disabled  AWVariant=Passthrough  PCopyVariant=Disabled  TRVariant=Disabled  FdbkBlocksVariant=Forward  IdealPFdbkVariant=Disabled  SatFdbkVariant=Disabled  DerivativeFilterVariant=ContFilter  NVariant=InternalParameters  NCopyVariant=Disabled  FilterICVariant=InternalICsFilter  IntegratorICVariant=InternalICs  ExternalResetVariant=Disabled  TRSumVariant=Passthrough  SumFdbkVariant=Disabled  SumVariant=Sum_PID  TsampFilterVariant=InternalTs  TsampNgainVariant=Passthrough  TsampIntegralVariant=Passthrough  ExternalSaturationOutDataTypeStr=Inherit: Same as second input
  PS-Simulink Converter : nesl_utility/PS-Simulink Converter  PhysicalDomain=network_engine_domain  SubClassName=ps_output  LeftPortType=input  RightPortType=output  PseudoPeriodic=off  Frequencies=[]  Unit=inherit  AffineConversion=off
      settings: SourceProductBaseCode=PW,SS
  PS-Simulink Converter1 : nesl_utility/PS-Simulink Converter  PhysicalDomain=network_engine_domain  SubClassName=ps_output  LeftPortType=input  RightPortType=output  PseudoPeriodic=off  Frequencies=[]  Unit=inherit  AffineConversion=off
      settings: SourceProductBaseCode=PW,SS
  Product : Product
  Sensing Angle1 : Subsystem
      mask Display: disp('a')
  Shaft Angle 2 : Scope
      settings: RequirementInfo={} %GIDa_a9f62d41_abf3_4de2_b298_9dc07658160c
  Shaft Free End : fl_lib/Mechanical/Rotational Elements/Rotational Free End  RequirementInfo={} %GIDa_85dceb17_1633_4d17_8b21_6dd5c111e202  w_specify=off  w_priority=None  w=0 rad/s  w_nominal_specify=off  w_nominal_unit=rad/s  w_nominal_value=1
      settings: SourceProductBaseCode=SS
  Solver Configuration : nesl_utility/Solver Configuration  RequirementInfo={} %GIDa_6eeeab8f_a399_4e38_93b2_d52ecab3b1e1  PhysicalDomain=network_engine_domain  SubClassName=solver  LeftPortType=input  RightPortType=generic  Tones=[]  Harmonics=[]  SimulateNoise=off  Profile=off  UseLocalSampling=off  EnableSwitchedLinearOptims=on  FrequencyDomain=off  UseCCode=off  RelTol=0.001  AbsTol=1e-06  MinStep=1e-09  ToWorkspace=off  RevertToSquareIcSolve=off  NumHomotopyIterations=100  PhasorMode=off  PhasorModeNumHarmonics=1  DoDC=off  ResidualTolerance=1e-7  UseLocalSolver=off  LocalSolverChoice=NE_BACKWARD_EULER_ADVANCER  LocalSolverSampleTime=.001  DoFixedCost=off  MaxNonlinIter=3  MaxModeIter=2  ComputeImpulses=off  ImpulseIterations=2  LinearAlgebra=auto  EquationFormulation=NE_TIME_EF  DelaysMemoryBudget=1024  AutomaticFiltering=on  FilteringTimeConstant=0.001  PartitionStorageMethod=AS_NEEDED  PartitionMemoryBudget=1024  PartitionMethod=FAST
      settings: SourceProductBaseCode=PW,SS
  Stepper Motor Driver : ee_lib/Electromechanical/Reluctance & Stepper/Stepper Motor Driver  RequirementInfo={} %GIDa_b75ce1e9_7c8f_42f1_a15d_a0f62381b5fe  step_or_av=ee.enum.electromech.simulationMode.stepping  step_rate_per_volt=10 Hz/V  Venable=2.5 V  Vreverse=2.5 V  supply_ports=ee.enum.supply_ports.hidesupply  Vm=5 V  Vsupply=10 V  half_stepping=ee.enum.electromech.steppingModeAveraged.fullStep  stepping_mode=ee.enum.electromech.steppingMode.microStep  numMicroSteps=4  Im=1.2 A
      settings: SourceProductBaseCode=PS  InternalSimscapePortConfiguration="{\"Bottom\":[],\"Left\":[{\"id\":\"ENA\",\"label\":\"ENA\",\"type\":\"foundation.electrical.electrical\"},{\"id\":\"REF\",\"label\":\"REF\",\"type\":\"foundation.electrical.electrical\"},{\"id\":\"REV\",\"label\":\"REV\",\"type\":\"foundation.electrical.electrical\"}],\"Right\":[{\"id\":\"pA\",\"label\":\"A+\",\"type\":\"foundation.electrical.electrical\"},{\"id\":\"nA\",\"label\":\"A-\",\"type\":\"foundation.electrical.electrical\"},{\"id\":\"pB\",\"label\":\"B+\",\"type\":\"foundation.electrical.electrical\"},{\"id\":\"nB\",\"label\":\"B-\",\"type\":\"foundation.electrical.electrical\"}],\"Top\":[]}"
  Stepper Motor2 : ee_lib/Electromechanical/Reluctance & Stepper/Stepper Motor  RequirementInfo={} %GIDa_9b029210_31fb_41a4_84be_bc9d94f54386  step_or_av=ee.enum.electromech.simulationMode.stepping  Ra=0.76 Ohm  La=8.4 mH  Km=2.4 N*m/A  Td=0.065 N*m  Rm=Inf Ohm  w_vec=[ 0 1000 3e+3 ] rpm  T_vec=[ 2 2 1 ] N*m  assert_if_slipping=ee.enum.assertAction.none  J_total=1e-4 kg*m^2  max_step_rate=10 Hz  Step=1.8 deg  J=2700 g*cm^2  B=1e-02 N*m/(rad/s)  speed0=0 rpm  theta0=0 deg  alpha=[.00393, .00393] 1/K  Tmeas=25 degC  Tmeas2=125 degC  T_vec2=[1.7, 1.7, .85] N*m  half_stepping=ee.enum.electromech.steppingModeAveraged.fullStep  thermal_masses=[100, 100] J/K  initial_temperatures=[25, 25] degC  rotor_thermal_mass=50 J/K  rotor_initial_temperature=25 degC  Rm_percent_rotor=90
      settings: SourceProductBaseCode=PS  InternalSimscapePortConfiguration="{\"Bottom\":[],\"Left\":[{\"id\":\"pA\",\"label\":\"A+\",\"type\":\"foundation.electrical.electrical\"},{\"id\":\"nA\",\"label\":\"A-\",\"type\":\"foundation.electrical.electrical\"},{\"id\":\"pB\",\"label\":\"B+\",\"type\":\"foundation.electrical.electrical\"},{\"id\":\"nB\",\"label\":\"B-\",\"type\":\"foundation.electrical.electrical\"}],\"Right\":[{\"id\":\"R\",\"label\":\"R\",\"type\":\"foundation.mechanical.rotational.rotational\"},{\"id\":\"C\",\"label\":\"C\",\"type\":\"foundation.mechanical.rotational.rotational\"}],\"Top\":[]}"
  Sum : Sum  RequirementInfo={} %GIDa_4c038191_29bc_42bc_87f7_26541eec49ce  Inputs=|+-
  Voltage Sensor : fl_lib/Electrical/Electrical Sensors/Voltage Sensor
  power : Outport  RequirementInfo={} %GIDa_f7e0d458_d7ab_47c2_9f94_25f8b3d57d41
  wires:
  PID Controller/1 -> Controller/1(Ref)
  Sensing Angle1/1(theta) -> Delay One Step/1, Shaft Angle 2/1
  Sum/1 -> PID Controller/1
  In1/1 -> Sum/1
  Product/1 -> power/1
  PS-Simulink Converter1/1 -> Product/2
  PS-Simulink Converter/1 -> Product/1
  Delay One Step/1 -> Sum/2
  connections:
  Stepper Motor2/RConn1 -- Shaft Free End/LConn1 -- Sensing Angle1/LConn1 -- Friction Stepper 2/LConn1
  ERef B-/LConn1 -- Stepper Motor Driver/RConn4 -- Stepper Motor2/LConn4
  Controller/RConn3 -- Stepper Motor Driver/LConn3
  Mechanical Rotational Reference5/LConn1 -- Friction Stepper 2/RConn1
  Stepper Motor Driver/RConn3 -- Stepper Motor2/LConn3
  Stepper Motor Driver/RConn2 -- Voltage Sensor/RConn2 -- Stepper Motor2/LConn2 -- ERef A+/LConn1
  MRRef Motor/LConn1 -- Stepper Motor2/RConn2 -- Solver Configuration/RConn1
  Controller/RConn1 -- Stepper Motor Driver/LConn1
  Stepper Motor Driver/RConn1 -- Current Sensor/LConn1 -- Voltage Sensor/LConn1
  Controller/RConn2 -- Stepper Motor Driver/LConn2
  Voltage Sensor/RConn1 -- PS-Simulink Converter1/LConn1
  PS-Simulink Converter/LConn1 -- Current Sensor/RConn1
  Current Sensor/RConn2 -- Stepper Motor2/LConn1

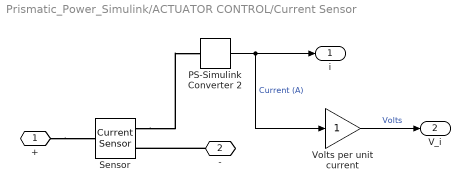
== system Prismatic_Power_Simulink/ACTUATOR CONTROL/Current Sensor ==
  PS-Simulink Converter 2 : nesl_utility/PS-Simulink Converter  RequirementInfo={} %GIDa_b597bef3_733c_403c_bcf9_0b1426886832  PhysicalDomain=network_engine_domain  SubClassName=ps_output  LeftPortType=input  RightPortType=output  PseudoPeriodic=off  Frequencies=[]  Unit=A  AffineConversion=off
      settings: SourceProductBaseCode=PW,SS
  Sensor : fl_lib/Electrical/Electrical Sensors/Current Sensor  RequirementInfo={} %GIDa_a4328683_2858_4231_9ac0_b08da630373c
  Volts per unit current : Gain  RequirementInfo={} %GIDa_29f53267_f9e5_465c_9d5e_f1bf25e897e2
  + : PMIOPort  RequirementInfo={} %GIDa_b3fced43_a7b6_47c0_b15c_d26a07a5e0c5  Side=Right
  - : PMIOPort  RequirementInfo={} %GIDa_096af8ce_0d67_44ca_b623_047ef1e17bc6  Port=2  Side=Left
  i : Outport  RequirementInfo={} %GIDa_cabbad7d_5123_4251_998c_4848aac354c3  VectorParamsAs1DForOutWhenUnconnected=off
  V_i : Outport  RequirementInfo={} %GIDa_eb44ef4a_6bc5_4b58_ad74_e0d7afc0d0cc  Port=2  VectorParamsAs1DForOutWhenUnconnected=off
  wires:
  PS-Simulink Converter 2/1 -> Volts per unit current/1, i/1  "Current (A)"
  Volts per unit current/1 -> V_i/1  "Volts"
  connections:
  +/RConn1 -- Sensor/LConn1
  -/RConn1 -- Sensor/RConn2
  Sensor/RConn1 -- PS-Simulink Converter 2/LConn1

== system Prismatic_Power_Simulink/ACTUATOR CONTROL/PWM Scope ==
  Electrical Reference1 : fl_lib/Electrical/Electrical Elements/Electrical Reference  RequirementInfo={} %GIDa_87969f43_0e6d_44f7_974c_6bbeb042b560
  PS-Simulink Converter 2 : nesl_utility/PS-Simulink Converter  RequirementInfo={} %GIDa_9e587847_c0d4_40d8_9091_e42d152db9e3  PhysicalDomain=network_engine_domain  SubClassName=ps_output  LeftPortType=input  RightPortType=output  PseudoPeriodic=off  Frequencies=[]  Unit=V  AffineConversion=off
      settings: SourceProductBaseCode=PW,SS
  PWM : Scope
      settings: RequirementInfo={} %GIDa_30cb1d91_1cbc_46d0_a7d4_8e9d2a6824c1
  Voltage Sensor : fl_lib/Electrical/Electrical Sensors/Voltage Sensor  RequirementInfo={} %GIDa_1b496ce4_7428_43a4_9638_48538f006573
  u : PMIOPort  RequirementInfo={} %GIDa_eb10fb5c_ec3d_443a_9d1c_ffa7fc75c909  Side=Left
  wires:
  PS-Simulink Converter 2/1 -> PWM/1
  connections:
  Voltage Sensor/RConn2 -- Electrical Reference1/LConn1
  Voltage Sensor/RConn1 -- PS-Simulink Converter 2/LConn1
  u/RConn1 -- Voltage Sensor/LConn1

== system Prismatic_Power_Simulink/ACTUATOR CONTROL/REV Scope ==
  Electrical Reference1 : fl_lib/Electrical/Electrical Elements/Electrical Reference  RequirementInfo={} %GIDa_1813bf2d_bb55_49c8_99b0_fd396f8a0391
  PS-Simulink Converter 2 : nesl_utility/PS-Simulink Converter  RequirementInfo={} %GIDa_8d949384_9e1e_4d5a_9f20_e7c7f97f7573  PhysicalDomain=network_engine_domain  SubClassName=ps_output  LeftPortType=input  RightPortType=output  PseudoPeriodic=off  Frequencies=[]  Unit=V  AffineConversion=off
      settings: SourceProductBaseCode=PW,SS
  REV : Scope
      settings: RequirementInfo={} %GIDa_5cac3262_57f9_4c66_a5a8_027990b676c0
  Voltage Sensor : fl_lib/Electrical/Electrical Sensors/Voltage Sensor  RequirementInfo={} %GIDa_37e02fa2_91f5_46a8_ab66_87cac6a5caf3
  u : PMIOPort  RequirementInfo={} %GIDa_a55e6308_56c2_4a28_b727_f27de629b35a  Side=Left
  wires:
  PS-Simulink Converter 2/1 -> REV/1
  connections:
  Voltage Sensor/RConn2 -- Electrical Reference1/LConn1
  Voltage Sensor/RConn1 -- PS-Simulink Converter 2/LConn1
  u/RConn1 -- Voltage Sensor/LConn1

== system Prismatic_Power_Simulink/ACTUATOR CONTROL/Vr Scope ==
  Electrical Reference1 : fl_lib/Electrical/Electrical Elements/Electrical Reference  RequirementInfo={} %GIDa_f933da43_8181_4984_8267_b5880da11195
  PS-Simulink Converter 2 : nesl_utility/PS-Simulink Converter  RequirementInfo={} %GIDa_0077381b_6450_45af_900c_503f04853d48  PhysicalDomain=network_engine_domain  SubClassName=ps_output  LeftPortType=input  RightPortType=output  PseudoPeriodic=off  Frequencies=[]  Unit=V  AffineConversion=off
      settings: SourceProductBaseCode=PW,SS
  Voltage Sensor : fl_lib/Electrical/Electrical Sensors/Voltage Sensor  RequirementInfo={} %GIDa_45ddd4f9_1b63_4e78_bd6c_d516004d6ea2
  Vr : Scope
      settings: RequirementInfo={} %GIDa_8491e282_6d6d_4b0e_b3fd_3464b2f5fb2a
  u : PMIOPort  RequirementInfo={} %GIDa_73aa022b_a278_41be_9d29_9a1dfc40ab59  Side=Left
  wires:
  PS-Simulink Converter 2/1 -> Vr/1
  connections:
  u/RConn1 -- Voltage Sensor/LConn1
  Voltage Sensor/RConn1 -- PS-Simulink Converter 2/LConn1
  Voltage Sensor/RConn2 -- Electrical Reference1/LConn1

== system Prismatic_Power_Simulink/STEPPER 1 CONTROL/Controller1 ==
  Ref : Inport  RequirementInfo={} %GIDa_81f5b3fb_241e_40ab_99c9_75a2543e3471
  Position : Subsystem  RequirementInfo={} %GIDa_e9fb77b6_89da_4a4a_b09b_fb9a37a7d5d7  VariantControl=Position
  Speed : Subsystem  RequirementInfo={} %GIDa_2266dfc8_b201_4769_86c5_abab30e69c03  VariantControl=Speed
  PWM : PMIOPort  RequirementInfo={} %GIDa_2a0e45c8_ca3f_4c9e_8c4a_9f65c0ba7f3d  Side=Right
  0v : PMIOPort  RequirementInfo={} %GIDa_91d10215_2833_47d4_b89b_318f5a3fdd1a  Port=2  Side=Right
  REV : PMIOPort  RequirementInfo={} %GIDa_35ab49ce_2fbc_4ab8_a8aa_a95c8b79441a  Port=3  Side=Right

== system Prismatic_Power_Simulink/STEPPER 1 CONTROL/Sensing Angle1 ==
  MRRef : fl_lib/Mechanical/Rotational Elements/Mechanical Rotational Reference  RequirementInfo={} %GIDa_ebac26c7_6c21_4bb9_9489_d5ff1226857c
  Motion Sensor : fl_lib/Mechanical/Mechanical Sensors/Ideal Rotational Motion Sensor  RequirementInfo={} %GIDa_94294d97_acf7_4442_8a86_41197765ef36  wrap_angle=simscape.enum.onoff.off  offset=0 rad
  deg : nesl_utility/PS-Simulink Converter  RequirementInfo={} %GIDa_5eb6b6ab_51ee_4205_b700_324edf83fcc9  PhysicalDomain=network_engine_domain  SubClassName=ps_output  LeftPortType=input  RightPortType=output  PseudoPeriodic=off  Frequencies=[]  Unit=deg  AffineConversion=off
      settings: SourceProductBaseCode=PW,SS
  R : PMIOPort  RequirementInfo={} %GIDa_4fa91bbe_f446_437b_b3f9_6519cdffadcd  Side=Left
  theta : Outport  RequirementInfo={} %GIDa_81ce2a69_f4ca_499f_8154_82ba52104045  VectorParamsAs1DForOutWhenUnconnected=off
  wires:
  deg/1 -> theta/1
  connections:
  R/RConn1 -- Motion Sensor/LConn1
  Motion Sensor/RConn3 -- deg/LConn1
  MRRef/LConn1 -- Motion Sensor/RConn1

== system Prismatic_Power_Simulink/STEPPER 2 CONTROL/Controller ==
  Ref : Inport  RequirementInfo={} %GIDa_2cf30e52_92fb_4404_a69e_00e76b079e6b
  Speed : Subsystem  RequirementInfo={} %GIDa_01df46f4_6625_4b0f_899a_e6eec7da7a3b  VariantControl=Speed
  PWM : PMIOPort  RequirementInfo={} %GIDa_dae52640_3e2a_45d9_a4f9_3e4b761ada2f  Side=Right
  0v : PMIOPort  RequirementInfo={} %GIDa_8f477d1b_8f8d_43fb_a638_c843d6cb4af3  Port=2  Side=Right
  REV : PMIOPort  RequirementInfo={} %GIDa_03874e01_d02b_4f09_9256_bb6212f8df33  Port=3  Side=Right

== system Prismatic_Power_Simulink/STEPPER 2 CONTROL/Sensing Angle1 ==
  MRRef : fl_lib/Mechanical/Rotational Elements/Mechanical Rotational Reference
  Motion Sensor : fl_lib/Mechanical/Mechanical Sensors/Ideal Rotational Motion Sensor  wrap_angle=simscape.enum.onoff.off  offset=0 rad
  deg : nesl_utility/PS-Simulink Converter  PhysicalDomain=network_engine_domain  SubClassName=ps_output  LeftPortType=input  RightPortType=output  PseudoPeriodic=off  Frequencies=[]  Unit=deg  AffineConversion=off
      settings: SourceProductBaseCode=PW,SS
  R : PMIOPort  Side=Left
  theta : Outport  VectorParamsAs1DForOutWhenUnconnected=off
  wires:
  deg/1 -> theta/1
  connections:
  R/RConn1 -- Motion Sensor/LConn1
  Motion Sensor/RConn3 -- deg/LConn1
  MRRef/LConn1 -- Motion Sensor/RConn1

== system Prismatic_Power_Simulink/STEPPER 1 CONTROL/Controller1/Position ==
  Ref : Inport  RequirementInfo={} %GIDa_42ee3971_91a4_4691_830a_0e384f3266e5
  Algorithm and Pulse Generation : Subsystem  RequirementInfo={} %GIDa_6fdfff51_1092_4775_aa7b_5355a99ffb6d
  ERef : fl_lib/Electrical/Electrical Elements/Electrical Reference  RequirementInfo={} %GIDa_8f837fa2_f463_48b5_8a5b_87d55d5a9264
  PWM : PMIOPort  RequirementInfo={} %GIDa_683c4f40_d3e1_409f_9af0_cd0a34111d80  Side=Right
  0v : PMIOPort  RequirementInfo={} %GIDa_e3f85af6_096c_4da0_9c90_7ad3a481c6d5  Port=2  Side=Right
  REV : PMIOPort  RequirementInfo={} %GIDa_47231603_f10e_4479_ad1b_50e358592944  Port=3  Side=Right
  wires:
  Ref/1 -> Algorithm and Pulse Generation/1(Reference)
  connections:
  Algorithm and Pulse Generation/RConn2 -- PWM/RConn1
  Algorithm and Pulse Generation/RConn1 -- REV/RConn1
  ERef/LConn1 -- 0v/RConn1

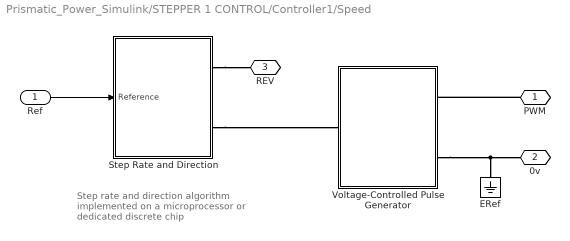
== system Prismatic_Power_Simulink/STEPPER 1 CONTROL/Controller1/Speed ==
  note: Step rate and direction algorithm implemented on a microprocessor or dedicated discrete chip
  Ref : Inport  RequirementInfo={} %GIDa_9a2b27ac_c09a_4978_b1ad_d4604276271d
  ERef : fl_lib/Electrical/Electrical Elements/Electrical Reference  RequirementInfo={} %GIDa_587e85ff_2581_47e3_9612_d0b63f998d53
  Step Rate and Direction : Subsystem  RequirementInfo={} %GIDa_2a1f1f64_a5ec_4214_8265_736170702319
  Voltage-Controlled Pulse Generator : Subsystem  RequirementInfo={} %GIDa_153dfaaf_1cad_44ec_977d_3f8775b676c4
  PWM : PMIOPort  RequirementInfo={} %GIDa_16360a7f_e273_4ab1_baa1_64cd9c89d02b  Side=Right
  0v : PMIOPort  RequirementInfo={} %GIDa_f1a818b0_9f01_46e7_bee6_5e13ba646be1  Port=2  Side=Right
  REV : PMIOPort  RequirementInfo={} %GIDa_8e05720b_f01d_4549_b9fa_21d8fac440b5  Port=3  Side=Right
  wires:
  Ref/1 -> Step Rate and Direction/1(Reference)
  connections:
  PWM/RConn1 -- Voltage-Controlled Pulse Generator/RConn1
  Voltage-Controlled Pulse Generator/RConn2 -- 0v/RConn1 -- ERef/LConn1
  Step Rate and Direction/RConn1 -- REV/RConn1
  Step Rate and Direction/RConn2 -- Voltage-Controlled Pulse Generator/LConn1

== system Prismatic_Power_Simulink/STEPPER 2 CONTROL/Controller/Speed ==
  Ref : Inport  RequirementInfo={} %GIDa_1a146f96_4770_40d7_a0ec_fb626119ae74
  ERef : fl_lib/Electrical/Electrical Elements/Electrical Reference  RequirementInfo={} %GIDa_5a87ed4d_0004_49a0_961e_0ad3ba0084c9
  Step Rate and Direction : Subsystem  RequirementInfo={} %GIDa_b055551f_d498_4a95_9fd0_1c5df64e37e3
  Voltage-Controlled Pulse Generator : Subsystem  RequirementInfo={} %GIDa_232f40c2_a31b_4da3_b0b2_2e563a7d0ff1
  PWM : PMIOPort  RequirementInfo={} %GIDa_372ffc4b_24b2_466f_9a5b_55af60aa4393  Side=Right
  0v : PMIOPort  RequirementInfo={} %GIDa_d45e4387_aca3_4e1a_8c42_30d7c4b6bd99  Port=2  Side=Right
  REV : PMIOPort  RequirementInfo={} %GIDa_239d32b8_b764_4af1_8fff_6791d906cadd  Port=3  Side=Right
  wires:
  Ref/1 -> Step Rate and Direction/1(Reference)
  connections:
  PWM/RConn1 -- Voltage-Controlled Pulse Generator/RConn1
  Voltage-Controlled Pulse Generator/RConn2 -- 0v/RConn1 -- ERef/LConn1
  Step Rate and Direction/RConn1 -- REV/RConn1
  Step Rate and Direction/RConn2 -- Voltage-Controlled Pulse Generator/LConn1

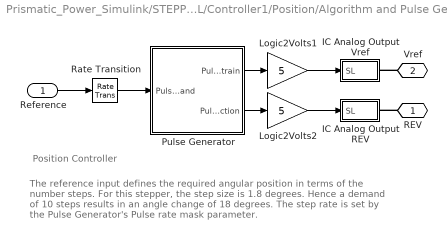
== system Prismatic_Power_Simulink/STEPPER 1 CONTROL/Controller1/Position/Algorithm and Pulse Generation ==
  note: The reference input defines the required angular position in terms of
      | the number steps. For this stepper, the step size is 1.8 degrees. Hence
      | a demand of 10 steps results in an angle change of 18 degrees.
      | The step rate is set by the Pulse Generator's Pulse rate mask parameter.
  note: Position Controller
  Reference : Inport  RequirementInfo={} %GIDa_bc15d19c_1d48_4998_96e9_208d8b8f7794
  IC Analog Output REV : Subsystem  RequirementInfo={} %GIDa_6cfc646c_426c_4d8c_8c88_0fa77f7a0858
  IC Analog Output Vref : Subsystem  RequirementInfo={} %GIDa_b5886147_7019_4d40_b4bf_a6840baf558c
  Logic2Volts1 : Gain  RequirementInfo={} %GIDa_f338c6f0_f929_4665_9723_f5f9d07ef2d4  Gain=5
  Logic2Volts2 : Gain  RequirementInfo={} %GIDa_eef83d19_99ad_4f10_a568_ab80f220af77  Gain=5
  Pulse Generator : Subsystem  RequirementInfo={} %GIDa_c2a491fe_5824_435c_af34_b8819ef8496a  mask{f=20}
      mask prompts: f "Pulse rate"
  Rate Transition : RateTransition  RequirementInfo={} %GIDa_d5c3b6c0_03a7_44ea_b1e8_ed5958021304  Deterministic=off
  REV : PMIOPort  RequirementInfo={} %GIDa_e6e3cceb_fc92_46d9_a04a_899fa64d40ce  Side=Right
  Vref : PMIOPort  RequirementInfo={} %GIDa_c2c31914_4b9f_442f_9594_84f371b796fa  Port=2  Side=Right
  wires:
  Logic2Volts1/1 -> IC Analog Output Vref/1(SL)
  Pulse Generator/1(Pulse train) -> Logic2Volts1/1
  Reference/1 -> Rate Transition/1
  Logic2Volts2/1 -> IC Analog Output REV/1(SL)
  Pulse Generator/2(Pulse direction) -> Logic2Volts2/1
  Rate Transition/1 -> Pulse Generator/1(Pulse  demand)
  connections:
  Vref/RConn1 -- IC Analog Output Vref/RConn1
  REV/RConn1 -- IC Analog Output REV/RConn1
